simulink model "ETCmodel_ver1"  (R2020b)
settings: Solver=VariableStepAuto  StartTime=0.0  StopTime=2  FixedStep=0.001  MaxStep=0.001  RelTol=1e-3  EnableMultiTasking=on
StopFcn:
  | ee_addSimlogTimeStamp(bdroot)
libraries: fl_lib x17, ee_lib x12, nesl_utility x12, arduinolib x4, eeQuadratureDecoder x1
CloseFcn:
  | try,close(h1_ee_motor_stepper),end
  | clear h1_ee_motor_stepper
  | try,close(h2_ee_motor_stepper),end
  | clear h2_ee_motor_stepper
  | 
  | clear simlog_ee_motor_stepper
  | clear logsout_ee_motor_stepper
  | clear RPM2 tout
Description:
  | Stepper Motor with Control
settings Model: Creator=The MathWorks, Inc.  LastModifiedBy=karto
settings DataIOCC: MaxDataPoints=10000  SaveFormat=Array  ReturnWorkspaceOutputs=off  SignalLoggingName=logsout_ee_motor_stepper
settings OptimizationCC: ExpressionDepthLimit=2147483647  InitFltsAndDblsToZero=on  LifeSpan=inf
settings DebuggingCC: UnderspecifiedInitializationDetection=Classic  MergeDetectMultiDrivingBlocksExec=none  FcnCallInpInsideContextMsg=warning  StateNameClashWarn=warning  SFUnexpectedBacktrackingDiag=warning  SFNoUnconditionalDefaultTransitionDiag=warning  SFExecutionAtInitializationDiag=none  ArithmeticOperatorsInVariantConditions=warning
settings HardwareCC: ProdBitPerPointer=32  ProdBitPerSizeT=32  ProdBitPerPtrDiffT=32  ProdLargestAtomicFloat=None  ProdIntDivRoundTo=Undefined  ProdEndianess=Unspecified  ProdWordSize=32  ProdHWDeviceType=32-bit Generic
settings ModelReferenceCC: PropagateSignalLabelsOutOfModel=off
settings SFSimCC: SimUseLocalCustomCode=off  CustomCodeUndefinedFunction=UseInterfaceOnly
settings RTWCC: RTWUseLocalCustomCode=off
settings CodeAppCC: StateflowObjectComments=on
settings GRTTargetCC: TargetLangStandard=C89/C90 (ANSI)  CombineOutputUpdateFcns=off  GRTInterface=on
settings ConfigComp: CovScope=ReferencedModels  CovMetricSettings=dw  CovSaveCumulativeToWorkspaceVar=on  CovSaveSingleToWorkspaceVar=on  CovExternalEMLEnable=off  CovSFcnEnable=off
settings SimscapeCC: SimscapeLogType=all  SimscapeLogSimulationStatistics=on  SimscapeLogName=simlog_ee_motor_stepper  SimscapeLogDataHistory=10000

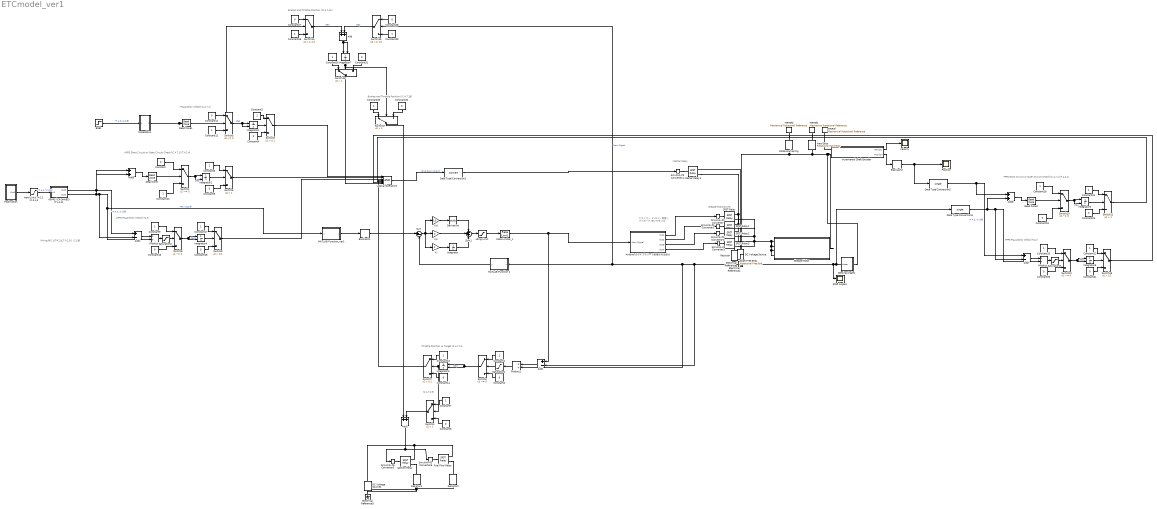
== system ETCmodel_ver1 ==
  note: ドライバー
      | ５V以下（駆動）
      | バイポーラ
      | 使いやすいの
  note: Brakes and Throttle Position (IC.4.7.1B)
  note: Brakes and Throttle Position (IC.4.7.1A)
  note: Throttle Position vs Target IC.4.7.2.A
  note: IC.4.7.2.B
  note: APPS Plausibility Check(T4.2)
  note: Wiring時にはT4.2.9_T.4.2.10に注意
  note: Master Relay
  note: APPS Short Circuit or Open Circuit Check(IC.4.7.1)(T.4.2.4)
  note: Plausibility Check(IC.4.7.1)
  note: StepperMotorDriver
  note: TPPS Plausibility Check(T4.2)
  note: TPPS Short Circuit or Open Circuit Check(IC.4.7.1)(T.4.2.4)
  AcPPS (CP-3HABS) (T.4.2.2) : Subsystem
  Add{,2..3,6} (4 alike) : Sum
  Add1 : Sum  Inputs=+-
  Add4 : Sum  Inputs=+-
  Add7 : Sum  Inputs=+-
  Arduinoのライブラリーで処理される部分 : Subsystem
  BSE1 : Step  SampleTime=0
  Backlash1 : Backlash  BacklashWidth=6  InitialOutput=511
  Backlash2 : Backlash  BacklashWidth=0.8  InitialOutput=511
  Constant{,2,4..5,8,11,14..16,19..21,23,27..28,31..32} (17 alike) : Constant  Value=0
  Constant{1,3,6..7,9..10,12..13,17..18,22,24..26,29..30,33} (17 alike) : Constant
  DC Voltage Source : fl_lib/Electrical/Electrical Sources/DC Voltage Source  v0=4.75 V
  DC Voltage Source1 : fl_lib/Electrical/Electrical Sources/DC Voltage Source  v0=12 V
  Data Type Conversion1 : DataTypeConversion  ConvertRealWorld=Stored Integer (SI)  LockScale=on
  Data Type Conversion2 : DataTypeConversion  OutDataTypeStr=single  ConvertRealWorld=Stored Integer (SI)  LockScale=on
  Data Type Conversion3 : DataTypeConversion  OutDataTypeStr=single  ConvertRealWorld=Stored Integer (SI)  LockScale=on
  Dead Zone : DeadZone  LowerValue=-1  UpperValue=1  SaturateOnIntegerOverflow=on
  Dead Zone1 : DeadZone  LowerValue=0.5  UpperValue=4.5  SaturateOnIntegerOverflow=on
  Dead Zone2 : DeadZone  LowerValue=-1  UpperValue=1  SaturateOnIntegerOverflow=on
  Derivative : Derivative
  Electrical Reference : fl_lib/Electrical/Electrical Elements/Electrical Reference
  Electrical Reference1 : fl_lib/Electrical/Electrical Elements/Electrical Reference
  Electrical Reference3 : fl_lib/Electrical/Electrical Elements/Electrical Reference
  Footmotion : Subsystem
  Fuel Flow Relay : ee_lib/Switches & Breakers/Relays/SPST Relay  block_choices=ee.enum.controlport.ps  R_closed=0.01 Ohm  G_open=1e-8 1/Ohm  Threshold=0.5  exposemeasurement=ee.enum.exposemeasurement.hidden  T_brk_C_S=0 s  T_mak_C_S=0 s  V_rated=5 V  V_energize=75  V_deenergize=25  l_winding=0.08 H  r_winding=12.5 Ohm  g_winding=1e-9 1/Ohm  enable_faults=ee.enum.relays.enable.no  fault_action=ee.enum.relays.faultaction.none  fault_types=ee.enum.relays.faultTypes.winding  fault_condition_ps=ee.enum.relays.faultConditionSPSTps.csstuck  r_deg_closed_s=1e-9 Ohm  winding_tau_fault=1e-3 s  tau_fault=1e-3 s  enable_temporal_fault=ee.enum.relays.enable.no  t_fault_stick=1 s  t_fault_ComOpen=1 s  t_fault=1 s  enable_behavioral_fault=ee.enum.relays.enable.no  winding_max_permissible_voltage=inf V  n_fail_on_voltage=1  winding_max_permissible_current=inf A  max_permissible_current=inf A  t_fail_on_current=1 s
      settings: SourceProductBaseCode=PS  InternalSimscapePortConfiguration="{\"Bottom\":[],\"Left\":[{\"id\":\"PS\",\"label\":\"PS\",\"type\":\"input\"}],\"Right\":[{\"id\":\"S\",\"label\":\"S\",\"type\":\"foundation.electrical.electrical\"},{\"id\":\"COM\",\"label\":\"C\",\"type\":\"foundation.electrical.electrical\"}],\"Top\":[]}"
  Hard Limit T4.2.1 IC.3.1.3 : Saturate  UpperLimit=0.75  LowerLimit=0.75
  Hard Stop : fl_lib/Mechanical/Rotational Elements/Rotational Hard Stop  upper_bnd=90 deg  lower_bnd=15 deg  stiff_up=1e6 N*m/rad  stiff_low=1e6 N*m/rad  D_up=0.01 N*m/(rad/s)  D_low=0.01 N*m/(rad/s)  model=simscape.enum.hardstop.smooth  transition=0.001 rad  w_specify=off  w_priority=None  w=0 rad/s  w_nominal_specify=off  w_nominal_unit=rad/s  w_nominal_value=1  t_specify=off  t_priority=None  t=0 N*m  t_nominal_specify=off  t_nominal_unit=N*m  t_nominal_value=1  phi_specify=off  phi_priority=High  phi=0 rad  phi_nominal_specify=off  phi_nominal_unit=rad  phi_nominal_value=1
      settings: SourceProductBaseCode=SS
  Idling Limit : Saturate  UpperLimit=90  LowerLimit=15
  Ignition Relay : ee_lib/Switches & Breakers/Relays/SPST Relay  block_choices=ee.enum.controlport.ps  R_closed=0.01 Ohm  G_open=1e-8 1/Ohm  Threshold=0.5  exposemeasurement=ee.enum.exposemeasurement.hidden  T_brk_C_S=0 s  T_mak_C_S=0 s  V_rated=5 V  V_energize=75  V_deenergize=25  l_winding=0.08 H  r_winding=12.5 Ohm  g_winding=1e-9 1/Ohm  enable_faults=ee.enum.relays.enable.no  fault_action=ee.enum.relays.faultaction.none  fault_types=ee.enum.relays.faultTypes.winding  fault_condition_ps=ee.enum.relays.faultConditionSPSTps.csstuck  r_deg_closed_s=1e-9 Ohm  winding_tau_fault=1e-3 s  tau_fault=1e-3 s  enable_temporal_fault=ee.enum.relays.enable.no  t_fault_stick=1 s  t_fault_ComOpen=1 s  t_fault=1 s  enable_behavioral_fault=ee.enum.relays.enable.no  winding_max_permissible_voltage=inf V  n_fail_on_voltage=1  winding_max_permissible_current=inf A  max_permissible_current=inf A  t_fail_on_current=1 s
      settings: SourceProductBaseCode=PS  InternalSimscapePortConfiguration="{\"Bottom\":[],\"Left\":[{\"id\":\"PS\",\"label\":\"PS\",\"type\":\"input\"}],\"Right\":[{\"id\":\"S\",\"label\":\"S\",\"type\":\"foundation.electrical.electrical\"},{\"id\":\"COM\",\"label\":\"C\",\"type\":\"foundation.electrical.electrical\"}],\"Top\":[]}"
  Incremental Shaft Encoder : Subsystem
  Integrator : Integrator
  Integrator{1..7} (7 alike) : Integrator  ExternalReset=rising  WrappedStateUpperValue=1  WrappedStateLowerValue=0  ZeroCross=off
  Kd : Gain  Gain=1.5
  Ki : Gain
  Kp : Gain  Gain=2
  Logical Operator2 : Logic  Inputs=7  AllPortsSameDT=off  OutDataTypeStr=boolean
  MATLAB Function 2 : MATLAB Function  TreatAsAtomicUnit=on
  MATLAB Function_ver1 : MATLAB Function  TreatAsAtomicUnit=on
  MRRef : fl_lib/Mechanical/Rotational Elements/Mechanical Rotational Reference
      settings: SourceProductName=Foundation Library
  MRRef1 : fl_lib/Mechanical/Rotational Elements/Mechanical Rotational Reference
      settings: SourceProductName=Foundation Library
  MRRef2 : fl_lib/Mechanical/Rotational Elements/Mechanical Rotational Reference
      settings: SourceProductName=Foundation Library
  Master Relay1 : ee_lib/Switches & Breakers/Relays/SPST Relay  block_choices=ee.enum.controlport.ps  R_closed=0.01 Ohm  G_open=1e-8 1/Ohm  Threshold=0.5  exposemeasurement=ee.enum.exposemeasurement.hidden  T_brk_C_S=0 s  T_mak_C_S=0 s  V_rated=5 V  V_energize=75  V_deenergize=25  l_winding=0.08 H  r_winding=12.5 Ohm  g_winding=1e-9 1/Ohm  enable_faults=ee.enum.relays.enable.no  fault_action=ee.enum.relays.faultaction.none  fault_types=ee.enum.relays.faultTypes.winding  fault_condition_ps=ee.enum.relays.faultConditionSPSTps.csstuck  r_deg_closed_s=1e-9 Ohm  winding_tau_fault=1e-3 s  tau_fault=1e-3 s  enable_temporal_fault=ee.enum.relays.enable.no  t_fault_stick=1 s  t_fault_ComOpen=1 s  t_fault=1 s  enable_behavioral_fault=ee.enum.relays.enable.no  winding_max_permissible_voltage=inf V  n_fail_on_voltage=1  winding_max_permissible_current=inf A  max_permissible_current=inf A  t_fail_on_current=1 s
      settings: SourceProductBaseCode=PS  InternalSimscapePortConfiguration="{\"Bottom\":[],\"Left\":[{\"id\":\"PS\",\"label\":\"PS\",\"type\":\"input\"}],\"Right\":[{\"id\":\"S\",\"label\":\"S\",\"type\":\"foundation.electrical.electrical\"},{\"id\":\"COM\",\"label\":\"C\",\"type\":\"foundation.electrical.electrical\"}],\"Top\":[]}"
  MotecECU1 : Subsystem
  Position : Scope
  Product1 : Product  Inputs=*/
  Product2 : Product  Inputs=*/
  Product3 : Product  Inputs=*/
  Rate Limiter_1 : RateLimiter  RisingSlewLimit=80  FallingSlewLimit=-100
  Resistor : ee_lib/Passive/Resistor  R=1 kOhm  R_tol=5  enable_R_tol=0  tol_distribution=1  nSigma=4  enable_operating_limits=0  operating_limit_action=2  max_working_voltage=100 V  power_rating=1 W  enable_faults=0  fault_action=1  R_faulted=inf Ohm  enable_temporal_fault=0  t_fault=1 s  enable_behavioral_fault=0  max_permissible_current=1 A  t_fail_on_current=1 s  noise_mode=0  sample_time=1e-3 s  repeatability=1  auto_seed=2531915367  user_seed=0  Tdevice=25 degC  alpha=3.93e-3 1/K  Tmeas=25 degC  thermal_mass=100 J/K  power_derating_T1=70 degC  power_derating_T2=155 degC  operating_temperature_range_vec=[-50, 150] degC  temperature_specify=off  temperature_priority=High  temperature=298.15 K  temperature_nominal_specify=off  temperature_nominal_unit=K  temperature_nominal_value=1
  Resistor1 : ee_lib/Passive/Resistor  R=1 kOhm  R_tol=5  enable_R_tol=0  tol_distribution=1  nSigma=4  enable_operating_limits=0  operating_limit_action=2  max_working_voltage=100 V  power_rating=1 W  enable_faults=0  fault_action=1  R_faulted=inf Ohm  enable_temporal_fault=0  t_fault=1 s  enable_behavioral_fault=0  max_permissible_current=1 A  t_fail_on_current=1 s  noise_mode=0  sample_time=1e-3 s  repeatability=1  auto_seed=1129453067  user_seed=0  Tdevice=25 degC  alpha=3.93e-3 1/K  Tmeas=25 degC  thermal_mass=100 J/K  power_derating_T1=70 degC  power_derating_T2=155 degC  operating_temperature_range_vec=[-50, 150] degC  temperature_specify=off  temperature_priority=High  temperature=298.15 K  temperature_nominal_specify=off  temperature_nominal_unit=K  temperature_nominal_value=1
  Resistor2 : ee_lib/Passive/Resistor  R=1 kOhm  R_tol=5  enable_R_tol=0  tol_distribution=1  nSigma=4  enable_operating_limits=0  operating_limit_action=2  max_working_voltage=100 V  power_rating=1 W  enable_faults=0  fault_action=1  R_faulted=inf Ohm  enable_temporal_fault=0  t_fault=1 s  enable_behavioral_fault=0  max_permissible_current=1 A  t_fail_on_current=1 s  noise_mode=0  sample_time=1e-3 s  repeatability=1  auto_seed=3511338023  user_seed=0  Tdevice=25 degC  alpha=3.93e-3 1/K  Tmeas=25 degC  thermal_mass=100 J/K  power_derating_T1=70 degC  power_derating_T2=155 degC  operating_temperature_range_vec=[-50, 150] degC  temperature_specify=off  temperature_priority=High  temperature=298.15 K  temperature_nominal_specify=off  temperature_nominal_unit=K  temperature_nominal_value=1
  Rotational Spring : fl_lib/Mechanical/Rotational Elements/Rotational Spring  spr_rate=10 N*m/rad  w_specify=off  w_priority=None  w=0 rad/s  w_nominal_specify=off  w_nominal_unit=rad/s  w_nominal_value=1  t_specify=off  t_priority=None  t=0 N*m  t_nominal_specify=off  t_nominal_unit=N*m  t_nominal_value=1  phi_specify=off  phi_priority=High  phi=0 rad  phi_nominal_specify=off  phi_nominal_unit=rad  phi_nominal_value=1
  SPST Relay{,1..3} (4 alike) : ee_lib/Switches & Breakers/Relays/SPST Relay  block_choices=ee.enum.controlport.ps  R_closed=0.01 Ohm  G_open=1e-8 1/Ohm  Threshold=0  exposemeasurement=ee.enum.exposemeasurement.hidden  T_brk_C_S=0 s  T_mak_C_S=0 s  V_rated=5 V  V_energize=75  V_deenergize=25  l_winding=0.08 H  r_winding=12.5 Ohm  g_winding=1e-9 1/Ohm  enable_faults=ee.enum.relays.enable.no  fault_action=ee.enum.relays.faultaction.none  fault_types=ee.enum.relays.faultTypes.winding  fault_condition_ps=ee.enum.relays.faultConditionSPSTps.csstuck  r_deg_closed_s=1e-9 Ohm  winding_tau_fault=1e-3 s  tau_fault=1e-3 s  enable_temporal_fault=ee.enum.relays.enable.no  t_fault_stick=1 s  t_fault_ComOpen=1 s  t_fault=1 s  enable_behavioral_fault=ee.enum.relays.enable.no  winding_max_permissible_voltage=inf V  n_fail_on_voltage=1  winding_max_permissible_current=inf A  max_permissible_current=inf A  t_fail_on_current=1 s
      settings: SourceProductBaseCode=PS  InternalSimscapePortConfiguration="{\"Bottom\":[],\"Left\":[{\"id\":\"PS\",\"label\":\"PS\",\"type\":\"input\"}],\"Right\":[{\"id\":\"S\",\"label\":\"S\",\"type\":\"foundation.electrical.electrical\"},{\"id\":\"COM\",\"label\":\"C\",\"type\":\"foundation.electrical.electrical\"}],\"Top\":[]}"
  Saturation1 : Saturate  UpperLimit=0.1  LowerLimit=-0.1
  Saturation2 : Saturate  UpperLimit=0.1  LowerLimit=-0.1
  Saturation3 : Saturate  UpperLimit=0.1  LowerLimit=-0.1
  Sensing Angle1 : Subsystem
  Shaft Angle1 : Scope
  Shaft Free End1 : fl_lib/Mechanical/Rotational Elements/Rotational Free End  w_specify=off  w_priority=None  w=0 rad/s  w_nominal_specify=off  w_nominal_unit=rad/s  w_nominal_value=1
      settings: SourceProductName=Foundation Library
  Simulink-PS Converter{,1..6} (7 alike) : nesl_utility/Simulink-PS Converter  PhysicalDomain=network_engine_domain  SubClassName=ps_input  LeftPortType=input  RightPortType=output  PseudoPeriodic=off  Frequencies=[]  NoiseDistribution=none  NoiseParameters=[]  Unit=1  AffineConversion=off  FilteringAndDerivatives=provide  SimscapeFilterOrder=1  InputFilterTimeConstant=0.001  UdotUserProvided=0
  StepperMotor : Subsystem
  Sum : Sum  Inputs=|+-
  Sum1 : Sum  Inputs=+++
  Switch{1..2,5,8,10,12} (6 alike) : Switch  Criteria=u2 ~= 0  InputSameDT=on
  Switch{4,6,11,16} (4 alike) : Switch  Criteria=u2 > Threshold  Threshold=1  InputSameDT=on
  Switch{3,7,9,13} (4 alike) : Switch  Criteria=u2 > Threshold  Threshold=0.1  InputSameDT=on
  Switch14 : Switch  Threshold=4.3  InputSameDT=on
  Switch15 : Switch  Threshold=4.3  InputSameDT=on
  Switch17 : Switch  Criteria=u2 > Threshold  Threshold=2  InputSameDT=on
  Velocity : Scope
  wires:
  Kd/1 -> Derivative/1
  Integrator/1 -> Sum1/3
  Sensing Angle1/1(theta) -> Switch15/2, MATLAB Function 2/1(u), Product1/2, Add1/2, Shaft Angle1/1, Data Type Conversion3/1  "Main Signal"
  Kp/1 -> Sum1/2
  Sum/1 -> Ki/1, Kd/1, Kp/1
  Ki/1 -> Integrator/1
  Sum1/1 -> Idling Limit/1
  Derivative/1 -> Sum1/1
  BSE1/1 -> MotecECU1/1(In1)  "*T.4.3.2に注意"
  Switch3/1 -> Logical Operator2/1
  Constant11/1 -> Switch5/1
  Switch5/1 -> Integrator1/2, Integrator1/1  "step"
  Constant12/1 -> Switch5/3
  Dead Zone1/1 -> Switch5/2
  AcPPS (CP-3HABS) (T.4.2.2)/2(Out1) -> MATLAB Function_ver1/1(u), Product2/2, Add4/2, Add3/2  "Main Signal"
  Switch6/1 -> Logical Operator2/2
  Dead Zone/1 -> Switch1/2
  AcPPS (CP-3HABS) (T.4.2.2)/1(Out2) -> Add4/1, Add3/1  "*T.4.2.7に注意"
  Constant10/1 -> Switch1/3
  Add3/1 -> Dead Zone/1
  Constant/1 -> Switch1/1
  Logical Operator2/1 -> Data Type Conversion1/1  "Shut Down Circuit"
  Idling Limit/1 -> Rate Limiter_1/1
  Data Type Conversion1/1 -> Simulink-PS Converter4/1
  Backlash1/1 -> Sum/1
  Backlash2/1 -> Data Type Conversion2/1, Position/1
  Arduinoのライブラリーで処理される部分/1(Out1) -> Simulink-PS Converter/1
  Arduinoのライブラリーで処理される部分/2(Out2) -> Simulink-PS Converter1/1
  Arduinoのライブラリーで処理される部分/3(Out3) -> Simulink-PS Converter2/1
  Arduinoのライブラリーで処理される部分/4(Out4) -> Simulink-PS Converter3/1
  Incremental Shaft Encoder/1(Velocity) -> Velocity/1
  Incremental Shaft Encoder/2(Position) -> Backlash2/1
  Rate Limiter_1/1 -> Add1/1, Arduinoのライブラリーで処理される部分/1(Main Signal)
  Integrator1/1 -> Switch3/2
  Constant3/1 -> Switch3/1
  Constant4/1 -> Switch3/3
  Switch1/1 -> Integrator2/1, Integrator2/2  "step"
  Integrator2/1 -> Switch6/2
  Constant6/1 -> Switch6/1
  Constant5/1 -> Switch6/3
  Constant9/1 -> Switch8/1
  Integrator4/1 -> Switch9/2
  Add4/1 -> Product2/1
  Constant17/1 -> Switch9/1
  Constant15/1 -> Switch8/3
  Constant16/1 -> Switch9/3
  Product2/1 -> Saturation2/1
  Switch8/1 -> Integrator4/2, Integrator4/1  "step"
  Saturation2/1 -> Switch8/2
  Switch9/1 -> Logical Operator2/3
  Switch13/1 -> Logical Operator2/6
  Saturation3/1 -> Switch12/2
  Switch12/1 -> Integrator6/1, Integrator6/2  "step"
  Product3/1 -> Saturation3/1
  Constant21/1 -> Switch13/3
  Constant20/1 -> Switch12/3
  Constant22/1 -> Switch13/1
  Add7/1 -> Product3/1
  Integrator6/1 -> Switch13/2
  Constant25/1 -> Switch12/1
  Constant23/1 -> Switch11/3
  Constant24/1 -> Switch11/1
  Integrator5/1 -> Switch11/2
  Switch10/1 -> Integrator5/2, Integrator5/1  "step"
  Constant18/1 -> Switch10/1
  Add6/1 -> Dead Zone2/1
  Constant19/1 -> Switch10/3
  Data Type Conversion2/1 -> Add7/1, Add6/1  "*T.4.2.7に注意"
  Dead Zone2/1 -> Switch10/2
  Switch11/1 -> Logical Operator2/5
  Data Type Conversion3/1 -> Add7/2, Product3/2, Add6/2
  Constant7/1 -> Switch4/1
  Constant8/1 -> Switch4/3
  Switch7/1 -> Logical Operator2/4
  Integrator3/1 -> Switch4/2, Switch7/2
  Add1/1 -> Product1/1
  Constant13/1 -> Switch7/1
  Product1/1 -> Saturation1/1
  Constant14/1 -> Switch7/3
  Saturation1/1 -> Switch2/2
  Constant2/1 -> Switch2/3
  Constant1/1 -> Switch2/1
  Switch2/1 -> Integrator3/2, Integrator3/1  "step"
  Switch4/1 -> Add2/2
  Add2/1 -> Simulink-PS Converter6/1, Simulink-PS Converter5/1
  Switch16/1 -> Logical Operator2/7
  MotecECU1/1(Out1) -> Switch14/2, Dead Zone1/1
  Constant27/1 -> Switch14/1
  Switch14/1 -> Add/1  "step"
  Constant29/1 -> Switch15/3
  Constant26/1 -> Switch14/3
  Switch15/1 -> Add/2  "step"
  Add/1 -> Integrator7/2, Integrator7/1
  Constant28/1 -> Switch15/1
  Constant31/1 -> Switch16/3
  Constant30/1 -> Switch16/1
  Switch17/1 -> Add2/1
  Integrator7/1 -> Switch17/2, Switch16/2
  Constant32/1 -> Switch17/3
  Constant33/1 -> Switch17/1
  MATLAB Function_ver1/1(y) -> Backlash1/1
  MATLAB Function 2/1(y) -> Sum/2
  Footmotion/1(Out1) -> Hard Limit T4.2.1 IC.3.1.3/1
  Hard Limit T4.2.1 IC.3.1.3/1 -> AcPPS (CP-3HABS) (T.4.2.2)/1(In1)  "*T.4.2.7に注意"
  connections:
  Incremental Shaft Encoder/LConn1 -- MRRef/LConn1
  StepperMotor/LConn2 -- StepperMotor/LConn3 -- StepperMotor/LConn4 -- SPST Relay/RConn2 -- SPST Relay1/RConn2 -- SPST Relay2/RConn2 -- Resistor/LConn1 -- SPST Relay3/RConn2 -- StepperMotor/LConn1
  Shaft Free End1/LConn1 -- Rotational Spring/LConn1 -- Hard Stop/LConn1 -- Sensing Angle1/LConn1 -- Incremental Shaft Encoder/LConn2 -- StepperMotor/RConn1
  Simulink-PS Converter3/RConn1 -- SPST Relay3/LConn1
  SPST Relay2/LConn1 -- Simulink-PS Converter2/RConn1
  Electrical Reference/LConn1 -- DC Voltage Source/RConn1
  SPST Relay/RConn1 -- Master Relay1/RConn2 -- SPST Relay3/RConn1 -- SPST Relay2/RConn1 -- SPST Relay1/RConn1
  Simulink-PS Converter/RConn1 -- SPST Relay/LConn1
  Simulink-PS Converter1/RConn1 -- SPST Relay1/LConn1
  Resistor/RConn1 -- Electrical Reference1/LConn1
  DC Voltage Source/LConn1 -- Master Relay1/RConn1
  Simulink-PS Converter4/RConn1 -- Master Relay1/LConn1
  DC Voltage Source1/LConn1 -- Fuel Flow Relay/RConn1 -- Ignition Relay/RConn1
  Electrical Reference3/LConn1 -- Resistor1/RConn1 -- Resistor2/RConn1 -- DC Voltage Source1/RConn1
  Ignition Relay/RConn2 -- Resistor1/LConn1
  Fuel Flow Relay/RConn2 -- Resistor2/LConn1
  Simulink-PS Converter5/RConn1 -- Ignition Relay/LConn1
  Simulink-PS Converter6/RConn1 -- Fuel Flow Relay/LConn1
  MRRef2/LConn1 -- Rotational Spring/RConn1
  MRRef1/LConn1 -- Hard Stop/RConn1

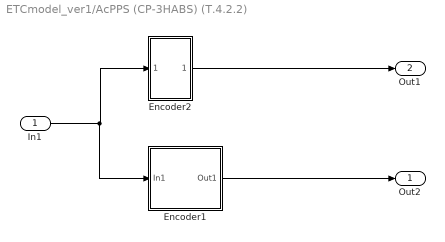
== system ETCmodel_ver1/AcPPS (CP-3HABS) (T.4.2.2) ==
  In1 : Inport
  Encoder1 : Subsystem
  Encoder2 : Subsystem
  Out2 : Outport
  Out1 : Outport  Port=2
  wires:
  In1/1 -> Encoder1/1(In1), Encoder2/1(In1)
  Encoder2/1(Out1) -> Out1/1
  Encoder1/1(Out1) -> Out2/1

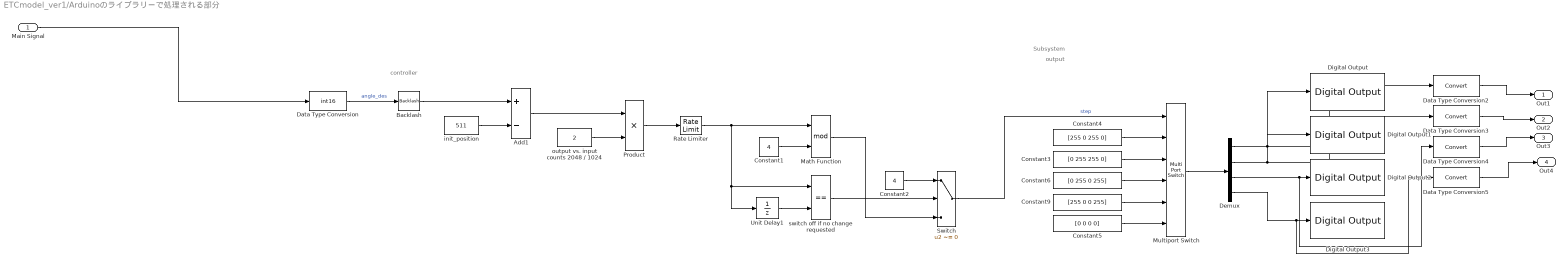
== system ETCmodel_ver1/Arduinoのライブラリーで処理される部分 ==
  note: Subsystem
  note: output
  note: controller
  Main Signal : Inport
  Add1 : Sum  Inputs=+-  InputSameDT=on
  Backlash : Backlash  BacklashWidth=6  InitialOutput=511
  Constant1 : Constant  Value=4  OutDataTypeStr=int16
  Constant2 : Constant  Value=4  OutDataTypeStr=int16
  Constant3 : Constant  Value=[0 255 255 0]  OutDataTypeStr=uint8
  Constant4 : Constant  Value=[255 0 255 0]  OutDataTypeStr=uint8
  Constant5 : Constant  Value=[0 0 0 0]  OutDataTypeStr=uint8
  Constant6 : Constant  Value=[0 255 0 255]  OutDataTypeStr=uint8
  Constant9 : Constant  Value=[255 0 0 255]  OutDataTypeStr=uint8
  Data Type Conversion : DataTypeConversion  OutDataTypeStr=int16
  Data Type Conversion{2..5} (4 alike) : DataTypeConversion
  Demux : Demux
  Digital Output : arduinolib/Digital Output  pinNumber=2  Direction=output  blockPlatform=arduino
  Digital Output1 : arduinolib/Digital Output  pinNumber=3  Direction=output  blockPlatform=arduino
  Digital Output2 : arduinolib/Digital Output  pinNumber=4  Direction=output  blockPlatform=arduino
  Digital Output3 : arduinolib/Digital Output  pinNumber=5  Direction=output  blockPlatform=arduino
  Math Function : Math  Operator=mod  SignedPower=on  SaturateOnIntegerOverflow=on
  Multiport Switch : MultiPortSwitch  DataPortOrder=Zero-based contiguous  Inputs=4  DataPortForDefault=Additional data port  DiagnosticForDefault=None  zeroidx=on  InputSameDT=on
  Product : Product  InputSameDT=on  OutDataTypeStr=int16  RndMeth=Zero
  Rate Limiter : RateLimiter  RisingSlewLimit=100  FallingSlewLimit=-100
  Switch : Switch  Criteria=u2 ~= 0  InputSameDT=on
  Unit Delay1 : UnitDelay  SampleTime=-1  HasFrameUpgradeWarning=on
  init_position : Constant  Value=511  OutDataTypeStr=int16
  output vs. input counts 2048 / 1024 : Constant  Value=2  OutDataTypeStr=int16
  switch off if no change requested : RelationalOperator  Operator===  OutDataTypeStr=boolean  RndMeth=Nearest  InputSameDT=on
  Out1 : Outport
  Out2 : Outport  Port=2
  Out3 : Outport  Port=3
  Out4 : Outport  Port=4
  wires:
  Rate Limiter/1 -> switch off if no change requested/1, Unit Delay1/1, Math Function/1
  Main Signal/1 -> Data Type Conversion/1
  Demux/2 -> Data Type Conversion3/1, Digital Output1/1
  Constant9/1 -> Multiport Switch/5
  Backlash/1 -> Add1/1
  Data Type Conversion/1 -> Backlash/1  "angle_des"
  Add1/1 -> Product/1
  Demux/1 -> Data Type Conversion2/1, Digital Output/1
  Data Type Conversion3/1 -> Out2/1
  Constant4/1 -> Multiport Switch/2
  output vs. input counts 2048 / 1024/1 -> Product/2
  Unit Delay1/1 -> switch off if no change requested/2
  Demux/3 -> Data Type Conversion4/1, Digital Output2/1
  Switch/1 -> Multiport Switch/1  "step"
  Multiport Switch/1 -> Demux/1
  Constant2/1 -> Switch/1
  Product/1 -> Rate Limiter/1
  Constant5/1 -> Multiport Switch/6
  Data Type Conversion4/1 -> Out3/1
  Math Function/1 -> Switch/3
  Constant3/1 -> Multiport Switch/3
  init_position/1 -> Add1/2
  switch off if no change requested/1 -> Switch/2
  Constant6/1 -> Multiport Switch/4
  Constant1/1 -> Math Function/2
  Data Type Conversion5/1 -> Out4/1
  Demux/4 -> Data Type Conversion5/1, Digital Output3/1
  Data Type Conversion2/1 -> Out1/1

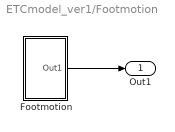
== system ETCmodel_ver1/Footmotion ==
  Footmotion : Subsystem
  Out1 : Outport
  wires:
  Footmotion/1(Out1) -> Out1/1

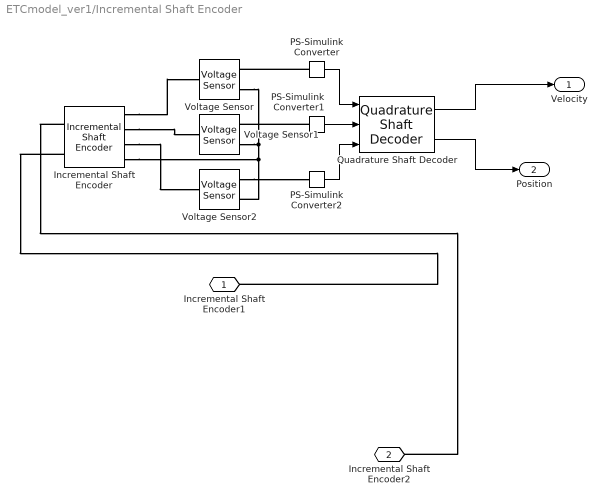
== system ETCmodel_ver1/Incremental Shaft Encoder ==
  Incremental Shaft Encoder : ee_lib/Sensors & Transducers/Incremental Shaft Encoder  NPulse=2  Vm=5 V  angle0=0 deg
      settings: SourceProductBaseCode=PS  InternalSimscapePortConfiguration="{\"Bottom\":[],\"Left\":[{\"id\":\"R\",\"label\":\"R\",\"type\":\"foundation.mechanical.rotational.rotational\"},{\"id\":\"C\",\"label\":\"C\",\"type\":\"foundation.mechanical.rotational.rotational\"}],\"Right\":[{\"id\":\"A\",\"label\":\"A\",\"type\":\"foundation.electrical.electrical\"},{\"id\":\"B\",\"label\":\"B\",\"type\":\"foundation.electrical.electrical\"},{\"id\":\"Z\",\"label\":\"Z\",\"type\":\"foundation.electrical.electrical\"},{\"id\":\"GND\",\"label\":\"REF\",\"type\":\"foundation.electrical.electrical\"}],\"Top\":[]}"
  PS-Simulink Converter : nesl_utility/PS-Simulink Converter  PhysicalDomain=network_engine_domain  SubClassName=ps_output  LeftPortType=input  RightPortType=output  PseudoPeriodic=off  Frequencies=[]  Unit=inherit  AffineConversion=off
  PS-Simulink Converter1 : nesl_utility/PS-Simulink Converter  PhysicalDomain=network_engine_domain  SubClassName=ps_output  LeftPortType=input  RightPortType=output  PseudoPeriodic=off  Frequencies=[]  Unit=inherit  AffineConversion=off
  PS-Simulink Converter2 : nesl_utility/PS-Simulink Converter  PhysicalDomain=network_engine_domain  SubClassName=ps_output  LeftPortType=input  RightPortType=output  PseudoPeriodic=off  Frequencies=[]  Unit=inherit  AffineConversion=off
  Quadrature Shaft Decoder : eeQuadratureDecoder/Quadrature Shaft Decoder  NPulse=200  Ts=0.5
      settings: SourceProductBaseCode=PS
  Voltage Sensor : fl_lib/Electrical/Electrical Sensors/Voltage Sensor
  Voltage Sensor1 : fl_lib/Electrical/Electrical Sensors/Voltage Sensor
  Voltage Sensor2 : fl_lib/Electrical/Electrical Sensors/Voltage Sensor
  Incremental Shaft Encoder1 : PMIOPort  Side=Left
  Incremental Shaft Encoder2 : PMIOPort  Port=2  Side=Left
  Velocity : Outport
  Position : Outport  Port=2
  wires:
  Quadrature Shaft Decoder/1 -> Velocity/1
  PS-Simulink Converter2/1 -> Quadrature Shaft Decoder/3
  PS-Simulink Converter1/1 -> Quadrature Shaft Decoder/2
  PS-Simulink Converter/1 -> Quadrature Shaft Decoder/1
  Quadrature Shaft Decoder/2 -> Position/1
  connections:
  Incremental Shaft Encoder/LConn2 -- Incremental Shaft Encoder1/RConn1
  Voltage Sensor1/RConn2 -- Incremental Shaft Encoder/RConn4 -- Voltage Sensor2/RConn2 -- Voltage Sensor/RConn2
  Incremental Shaft Encoder/RConn2 -- Voltage Sensor1/LConn1
  PS-Simulink Converter1/LConn1 -- Voltage Sensor1/RConn1
  Incremental Shaft Encoder/RConn3 -- Voltage Sensor2/LConn1
  Voltage Sensor2/RConn1 -- PS-Simulink Converter2/LConn1
  Incremental Shaft Encoder/RConn1 -- Voltage Sensor/LConn1
  PS-Simulink Converter/LConn1 -- Voltage Sensor/RConn1
  Incremental Shaft Encoder/LConn1 -- Incremental Shaft Encoder2/RConn1

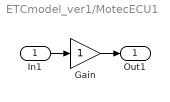
== system ETCmodel_ver1/MotecECU1 ==
  In1 : Inport
  Gain : Gain
  Out1 : Outport
  wires:
  Gain/1 -> Out1/1
  In1/1 -> Gain/1

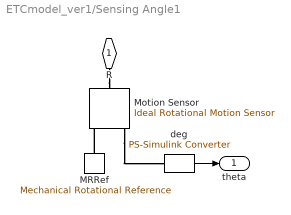
== system ETCmodel_ver1/Sensing Angle1 ==
  MRRef : fl_lib/Mechanical/Rotational Elements/Mechanical Rotational Reference
      settings: SourceProductName=Foundation Library
  Motion Sensor : fl_lib/Mechanical/Mechanical Sensors/Ideal Rotational Motion Sensor  wrap_angle=simscape.enum.onoff.off  offset=0 rad
      settings: SourceProductName=Foundation Library
  deg : nesl_utility/PS-Simulink Converter  PhysicalDomain=network_engine_domain  SubClassName=ps_output  LeftPortType=input  RightPortType=output  PseudoPeriodic=off  Frequencies=[]  Unit=deg  AffineConversion=off
      settings: SourceProductName=Utilities
  R : PMIOPort  Side=Left
  theta : Outport  VectorParamsAs1DForOutWhenUnconnected=off
  wires:
  deg/1 -> theta/1
  connections:
  R/RConn1 -- Motion Sensor/LConn1
  Motion Sensor/RConn3 -- deg/LConn1
  MRRef/LConn1 -- Motion Sensor/RConn1

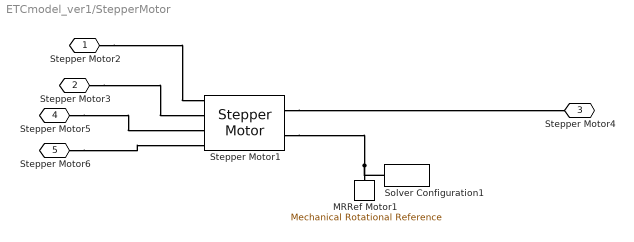
== system ETCmodel_ver1/StepperMotor ==
  MRRef Motor1 : fl_lib/Mechanical/Rotational Elements/Mechanical Rotational Reference
      settings: SourceProductName=Foundation Library
  Solver Configuration1 : nesl_utility/Solver Configuration  PhysicalDomain=network_engine_domain  SubClassName=solver  LeftPortType=input  RightPortType=generic  Tones=[]  Harmonics=[]  SimulateNoise=off  Profile=off  UseLocalSampling=off  EnableSwitchedLinearOptims=on  FrequencyDomain=off  UseCCode=off  RelTol=0.001  AbsTol=1e-06  MinStep=1e-09  ToWorkspace=off  RevertToSquareIcSolve=off  NumHomotopyIterations=100  PhasorMode=off  PhasorModeNumHarmonics=1  DoDC=off  ResidualTolerance=1e-9  UseLocalSolver=off  LocalSolverChoice=NE_BACKWARD_EULER_ADVANCER  LocalSolverSampleTime=.001  DoFixedCost=off  MaxNonlinIter=3  MaxModeIter=2  ComputeImpulses=off  ImpulseIterations=2  LinearAlgebra=auto  EquationFormulation=NE_TIME_EF  DelaysMemoryBudget=1024  AutomaticFiltering=on  FilteringTimeConstant=0.001  PartitionStorageMethod=AS_NEEDED  PartitionMemoryBudget=1024  PartitionMethod=FAST
      settings: SourceProductName=Utilities
  Stepper Motor1 : ee_lib/Electromechanical/Reluctance & Stepper/Stepper Motor  step_or_av=2  w_vec=[0, 1000, 3000] rpm  T_vec=[2, 2, 1] N*m  assert_if_slipping=0  J_total=1e-4 kg*m^2  max_step_rate=10 Hz  Ra=0.55 Ohm  La=1.5e-3 H  Km=0.19 N*m/A  Td=0 N*m  Rm=inf Ohm  Step=1.8 deg  J=4.5e-5 kg*m^2  B=8.0e-4 N*m/(rad/s)  speed0=0 rpm  theta0=0 deg  alpha=[.00393, .00393] 1/K  Tmeas=25 degC  T_vec2=[1.7, 1.7, .85] N*m  Tmeas2=125 degC  half_stepping=0  thermal_masses=[100, 100] J/K  initial_temperatures=[25, 25] degC  rotor_thermal_mass=50 J/K  rotor_initial_temperature=25 degC  Rm_percent_rotor=90
      settings: SourceProductBaseCode=PS  InternalSimscapePortConfiguration="{\"Bottom\":[],\"Left\":[{\"id\":\"pA\",\"label\":\"A+\",\"type\":\"foundation.electrical.electrical\"},{\"id\":\"nA\",\"label\":\"A-\",\"type\":\"foundation.electrical.electrical\"},{\"id\":\"pB\",\"label\":\"B+\",\"type\":\"foundation.electrical.electrical\"},{\"id\":\"nB\",\"label\":\"B-\",\"type\":\"foundation.electrical.electrical\"}],\"Right\":[{\"id\":\"R\",\"label\":\"R\",\"type\":\"foundation.mechanical.rotational.rotational\"},{\"id\":\"C\",\"label\":\"C\",\"type\":\"foundation.mechanical.rotational.rotational\"}],\"Top\":[]}"
  Stepper Motor2 : PMIOPort  Side=Left
  Stepper Motor3 : PMIOPort  Port=2  Side=Left
  Stepper Motor4 : PMIOPort  Port=3  Side=Right
  Stepper Motor5 : PMIOPort  Port=4  Side=Left
  Stepper Motor6 : PMIOPort  Port=5  Side=Left
  connections:
  MRRef Motor1/LConn1 -- Stepper Motor1/RConn2 -- Solver Configuration1/RConn1
  Stepper Motor3/RConn1 -- Stepper Motor1/LConn2
  Stepper Motor2/RConn1 -- Stepper Motor1/LConn1
  Stepper Motor1/RConn1 -- Stepper Motor4/RConn1
  Stepper Motor6/RConn1 -- Stepper Motor1/LConn4
  Stepper Motor5/RConn1 -- Stepper Motor1/LConn3

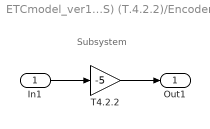
== system ETCmodel_ver1/AcPPS (CP-3HABS) (T.4.2.2)/Encoder1 ==
  note: Subsystem
  In1 : Inport
  T4.2.2 : Gain  Gain=-5
  Out1 : Outport
  wires:
  T4.2.2/1 -> Out1/1
  In1/1 -> T4.2.2/1

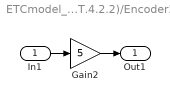
== system ETCmodel_ver1/AcPPS (CP-3HABS) (T.4.2.2)/Encoder2 ==
  In1 : Inport
  Gain2 : Gain  Gain=5
  Out1 : Outport
  wires:
  In1/1 -> Gain2/1
  Gain2/1 -> Out1/1

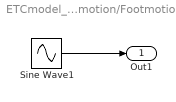
== system ETCmodel_ver1/Footmotion/Footmotion ==
  Sine Wave1 : Sin  SampleTime=0
  Out1 : Outport
  wires:
  Sine Wave1/1 -> Out1/1

== matlab function ETCmodel_ver1/MATLAB Function_ver1 ==
  data: u input; y output
function y = fcn(u)

y = u;

== matlab function ETCmodel_ver1/MATLAB Function 2 ==
  data: u input; y output
function y = fcn(u)

y = u;
